simulink model "spot410"  (R2024b)
settings: Solver=ode4  StartTime=0.0  StopTime=tsim  FixedStep=baseRate  RelTol=1e-6  AbsTol=1e-6
values from neighbouring files (symbols this model uses):
  baseRate = paramEst(phase,coord).k2    [SpotEstimator.m]
undefined symbols (not defined in the file or in its folder): a1, a2, a3, b0, b1, b2, b3, dataRate, DiscIntNeverNeededParam, drop_states_ARM, drop_states_BLACK, drop_states_BLUE, drop_states_RED, F_black_X_nominal, F_black_Y_nominal, F_blue_X_nominal, F_blue_Y_nominal, F_red_X_nominal, F_red_Y_nominal, F_thrusters_BLACK, F_thrusters_BLUE, F_thrusters_RED, Gamma1_el, Gamma1_sh, Gamma1_wr, Gamma2_el, Gamma2_sh, Gamma2_wr, Gamma3_el, Gamma3_sh, Gamma3_wr, Gamma4_el, Gamma4_sh, Gamma4_wr, Gamma5_el, Gamma5_sh, Gamma5_wr, Gamma6_el, Gamma6_sh, Gamma6_wr, home_states_BLACK, home_states_BLUE, home_states_RED, IBLACK, IBLUE, IDIST, IEE, init_states_BLACK, init_states_BLUE, init_states_RED, IPROX, IRED, K_BLACK, K_BLUE, K_RED, Kd_elarm, Kd_sharm, Kd_tb, Kd_tblue, Kd_tr ... (+49)
libraries: simulink x30, nvidiaSharedBlocks x19, MainLibrary x5, dspinverses x3, nvidiaIMUSensorslib x1
(part 7 of 7)

== matlab function spot410/Simulate Plant Dynamics/RED and ARM Dynamics/RED + ARM/Inertia Function 1 ==
  data: mRED parameter; IRED parameter; Phi parameter; b0 parameter; a1 parameter; b1 parameter; a2 parameter; b2 parameter; a3 parameter; b3 parameter; mPROX parameter; mDIST parameter; mEE parameter; IPROX parameter; IDIST parameter; InertiaS output; x input; IEE parameter
function InertiaS = InertiaFunc3LINK(mRED, IRED, Phi, b0, a1, b1, a2, b2, a3, b3, mPROX, mDIST, mEE, IPROX, IDIST, x, IEE)

    q0 = x(3);
    q1 = x(4);
    q2 = x(5);
    q3 = x(6);
    
    t2 = a1+b1;
    t3 = a1.*mPROX;
    t4 = mDIST.*t2;
    t5 = mEE.*t2;
    t6 = q0+q1;
    t7 = cos(t6);
    t8 = t3+t4+t5;
    t9 = a2.*mDIST;
    t10 = a2+b2;
    t11 = mEE.*t10;
    t12 = q0+q1+q2;
    t13 = cos(t12);
    t14 = t9+t11;
    t15 = q0+q1+q2+q3;
    t16 = cos(t15);
    t17 = mRED+mPROX+mDIST+mEE;
    t18 = b0.*mPROX;
    t19 = b0.*mDIST;
    t20 = b0.*mEE;
    t21 = t18+t19+t20;
    t22 = (pi/2-Phi)+q0;
    t23 = sin(t6);
    t24 = sin(t12);
    t25 = sin(t15);
    t26 = a2.*mEE;
    t27 = b2.*mEE;
    t28 = t9+t26+t27;
    t29 = sin(t22);
    t86 = t7.*t8;
    t87 = t13.*t14;
    t88 = a3.*mEE.*t16;
    t30 = -t86-t87-t88-t21.*t29;
    t31 = cos(t22);
    t32 = t21.*t31;
    t89 = t8.*t23;
    t90 = t14.*t24;
    t91 = a3.*mEE.*t25;
    t33 = t32-t89-t90-t91;
    t34 = a1.^2;
    t35 = a2.^2;
    t36 = b0.^2;
    t37 = b1.^2;
    t38 = a1.*a2.*mDIST.*2.0;
    t39 = a1.*a2.*mEE.*2.0;
    t40 = a2.*b1.*mDIST.*2.0;
    t41 = a1.*b2.*mEE.*2.0;
    t42 = a2.*b1.*mEE.*2.0;
    t43 = b1.*b2.*mEE.*2.0;
    t44 = t38+t39+t40+t41+t42+t43;
    t45 = cos(q2);
    t46 = t44.*t45;
    t47 = a2.*a3.*mEE.*2.0;
    t48 = a3.*b2.*mEE.*2.0;
    t49 = t47+t48;
    t50 = cos(q3);
    t51 = t49.*t50;
    t52 = a1.*a3.*mEE.*2.0;
    t53 = a3.*b1.*mEE.*2.0;
    t54 = t52+t53;
    t55 = q2+q3;
    t56 = cos(t55);
    t57 = t54.*t56;
    t58 = (pi/2-Phi)-q1;
    t59 = sin(t58);
    t60 = -(pi/2-Phi)+q1+q2;
    t61 = sin(t60);
    t62 = -(pi/2-Phi)+q1+q2+q3;
    t63 = sin(t62);
    t64 = mPROX.*t34;
    t65 = mDIST.*t34;
    t66 = mEE.*t34;
    t67 = mDIST.*t35;
    t68 = mEE.*t35;
    t69 = a3.^2;
    t70 = mEE.*t69;
    t71 = mDIST.*t37;
    t72 = mEE.*t37;
    t73 = b2.^2;
    t74 = mEE.*t73;
    t75 = a1.*b1.*mDIST.*2.0;
    t76 = a1.*b1.*mEE.*2.0;
    t77 = a2.*b2.*mEE.*2.0;
    t78 = a2.*b0.*mDIST;
    t79 = a2.*b0.*mEE;
    t80 = b0.*b2.*mEE;
    t81 = t78+t79+t80;
    t82 = a1.*a3.*mEE;
    t83 = a3.*b1.*mEE;
    t84 = t82+t83;
    t85 = t56.*t84;
    t92 = a1.*b0.*mPROX;
    t93 = a1.*b0.*mDIST;
    t94 = a1.*b0.*mEE;
    t95 = b0.*b1.*mDIST;
    t96 = b0.*b1.*mEE;
    t97 = t92+t93+t94+t95+t96;
    t98 = t59.*t97;
    t112 = t61.*t81;
    t113 = a3.*b0.*mEE.*t63;
    t99 = IPROX+IDIST+IEE+t46+t51+t57+t64+t65+t66+t67+t68+t70+t71+t72+t74+t75+t76+t77+t98-t112-t113;
    t100 = a1.*a2.*mDIST;
    t101 = a1.*a2.*mEE;
    t102 = a2.*b1.*mDIST;
    t103 = a1.*b2.*mEE;
    t104 = a2.*b1.*mEE;
    t105 = b1.*b2.*mEE;
    t106 = t100+t101+t102+t103+t104+t105;
    t107 = t45.*t106;
    t108 = a2.*a3.*mEE;
    t109 = a3.*b2.*mEE;
    t110 = t108+t109;
    t111 = t50.*t110;
    t114 = IDIST+IEE+t51+t67+t68+t70+t74+t77+t85+t107;
    t115 = IEE+t70+t85+t111;
    t116 = IEE+t70+t111;
    InertiaS = reshape([t17,0.0,t30,-t86-t87-t88,-t88-t13.*t28,-t88,0.0,t17,t33,-t89-t90-t91,-t91-t24.*t28,-t91,t30,t33,IRED+IPROX+IDIST+IEE+t46+t51+t57+t64+t65+t66+t67+t68+t70+t71+t72+t74+t75+t76+t77+t59.*(a1.*b0.*mPROX.*2.0+a1.*b0.*mDIST.*2.0+a1.*b0.*mEE.*2.0+b0.*b1.*mDIST.*2.0+b0.*b1.*mEE.*2.0)+mPROX.*t36+mDIST.*t36+mEE.*t36-t61.*(a2.*b0.*mDIST.*2.0+a2.*b0.*mEE.*2.0+b0.*b2.*mEE.*2.0)-a3.*b0.*mEE.*t63.*2.0,t99,IDIST+IEE+t51+t67+t68+t70+t74+t77+t85+t107-t112-t113,IEE+t70+t85+t111-t113,-t7.*t8-t13.*t14-a3.*mEE.*t16,-t8.*t23-t14.*t24-a3.*mEE.*t25,t99,IPROX+IDIST+IEE+t46+t51+t57+t64+t65+t66+t67+t68+t70+t71+t72+t74+t75+t76+t77,t114,t115,-t13.*t28-a3.*mEE.*t16,-t24.*t28-a3.*mEE.*t25,IDIST+IEE+t51+t67+t68+t70+t74+t77+t85+t107-t61.*t81-a3.*b0.*mEE.*t63,t114,IDIST+IEE+t51+t67+t68+t70+t74+t77,t116,-a3.*mEE.*t16,-a3.*mEE.*t25,IEE+t70+t85+t111-a3.*b0.*mEE.*t63,t115,t116,IEE+t70],[6,6]);
end

== matlab function spot410/Simulate Plant Dynamics/BLUE Dynamics/Calculated & Store Measured States/Subsystem1/Enabled Subsystem/MATLAB Function ==
  data: y input; dy output; dt input; tau input; dy_prev input; ema_prev input; ema output
function [dy, ema] = realtime_derivative_ema(y, dt, tau, dy_prev, ema_prev)
    % Inputs:
    % y: Current measurement
    % dt: Time step
    % alpha: Smoothing factor (e.g., 0.1)

    alpha = 1 - exp(-dt / tau);
        
    % Update EMA
    ema = alpha.*y + (1 - alpha).*ema_prev;
    
    % Compute derivative
    dy = (ema - ema_prev)./dt;
    
end

== matlab function spot410/Simulate Plant Dynamics/BLACK Dynamics/Dynamics Model for BLACK/MATLAB Function ==
  data: control_inputs input; x_ddot output; mBLACK parameter; IBLACK parameter
function x_ddot = BLACK_dynamics(control_inputs, mBLACK, IBLACK)

%#codegen
% Fully define the size of x_ddot() for code generation:
x_ddot     = zeros(3,1);

% Extract the control inputs from the control_input vector:
Fx        = control_inputs(1);              % [N]
Fy        = control_inputs(2);              % [N]
Tz        = control_inputs(3);              % [N.m]

% Calculate the state acceleration vector:
x_ddot(1) = Fx/mBLACK;                      % [m/s^2]
x_ddot(2) = Fy/mBLACK;                      % [m/s^2]
x_ddot(3) = Tz/IBLACK;                      % [rad/s^2]

end

== matlab function spot410/Simulate Plant Dynamics/BLUE Dynamics/BLUE  Dynamics Model/MATLAB Function ==
  data: control_inputs input; x_ddot output; mBLUE parameter; IBLUE parameter
function x_ddot = BLUE_dynamics(control_inputs, mBLUE, IBLUE)%#codegen
% Fully define the size of x_ddot() for code generation:
x_ddot     = zeros(3,1);

% Extract the control inputs from the control_input vector:
Fx        = control_inputs(1);              % [N]
Fy        = control_inputs(2);              % [N]
Tz        = control_inputs(3);              % [N.m]

% Calculate the state acceleration vector:
x_ddot(1) = Fx/mBLUE;                      % [m/s^2]
x_ddot(2) = Fy/mBLUE;                      % [m/s^2]
x_ddot(3) = Tz/IBLUE;                      % [rad/s^2]

end

== matlab function spot410/Gyro.//Accel. Code/Log Gyro//Accel/Parse IMU Data ==
  data: WhoAmI input; RED_IMU_Ax output; IMU_Ax input; IMU_Ay input; IMU_Gz input; RED_IMU_Ay output; RED_IMU_Gz output; BLACK_IMU_Ax output; BLACK_IMU_Ay output; BLACK_IMU_Gz output; BLUE_IMU_Ax output; BLUE_IMU_Ay output; BLUE_IMU_Gz output
function [RED_IMU_Ax, RED_IMU_Ay, RED_IMU_Gz, BLACK_IMU_Ax, BLACK_IMU_Ay, BLACK_IMU_Gz, BLUE_IMU_Ax, BLUE_IMU_Ay, BLUE_IMU_Gz] = ParseIMUData(WhoAmI, IMU_Ax, IMU_Ay, IMU_Gz)

    if WhoAmI == 1 % This is RED

        RED_IMU_Ax = IMU_Ax;
        RED_IMU_Ay = IMU_Ay;
        RED_IMU_Gz = IMU_Gz;
        BLACK_IMU_Ax = 0;
        BLACK_IMU_Ay = 0;
        BLACK_IMU_Gz = 0;
        BLUE_IMU_Ax = 0;
        BLUE_IMU_Ay = 0;
        BLUE_IMU_Gz = 0;

    elseif WhoAmI == 2 % This is BLACK

        RED_IMU_Ax = 0;
        RED_IMU_Ay = 0;
        RED_IMU_Gz = 0;
        BLACK_IMU_Ax = IMU_Ax;
        BLACK_IMU_Ay = IMU_Ay;
        BLACK_IMU_Gz = IMU_Gz;
        BLUE_IMU_Ax = 0;
        BLUE_IMU_Ay = 0;
        BLUE_IMU_Gz = 0;

    elseif WhoAmI == 3 % This is BLUE

        RED_IMU_Ax = 0;
        RED_IMU_Ay = 0;
        RED_IMU_Gz = 0;
        BLACK_IMU_Ax = 0;
        BLACK_IMU_Ay = 0;
        BLACK_IMU_Gz = 0;
        BLUE_IMU_Ax = IMU_Ax;
        BLUE_IMU_Ay = IMU_Ay;
        BLUE_IMU_Gz = IMU_Gz;

    else 

        RED_IMU_Ax = 0;
        RED_IMU_Ay = 0;
        RED_IMU_Gz = 0;
        BLACK_IMU_Ax = 0;
        BLACK_IMU_Ay = 0;
        BLACK_IMU_Gz = 0;
        BLUE_IMU_Ax = 0;
        BLUE_IMU_Ay = 0;
        BLUE_IMU_Gz = 0;       

    end

end

== matlab function spot410/Simulate Plant Dynamics/BLUE Dynamics/Calculated & Store Measured States/Subsystem2/Enabled Subsystem/MATLAB Function ==
  data: y input; dy output; dt input; tau input; dy_prev input; ema_prev input; ema output
function [dy, ema] = realtime_derivative_ema(y, dt, tau, dy_prev, ema_prev)
    % Inputs:
    % y: Current measurement
    % dt: Time step
    % alpha: Smoothing factor (e.g., 0.1)

    alpha = 1 - exp(-dt / tau);
        
    % Update EMA
    ema = alpha.*y + (1 - alpha).*ema_prev;
    
    % Compute derivative
    dy = (ema - ema_prev)./dt;
    
end

== matlab function spot410/Simulate Plant Dynamics/BLUE Dynamics/Data @ Measurement Rate/Calculate True Time Step/MATLAB Function ==
  data: dt input; dt_out output; dataRate input
function dt_out = CheckforInvalidTime(dt, dataRate)

    if dt <= 0

        dt_out = dataRate;

    else

        dt_out = dt;

    end


end

== matlab function spot410/SpotGnc/SpotCtrlErr ==
  data: phase input; ref input; ref_vel input; est input; est_vel input; err output; paramCtrlErr parameter; err_vel output
function [err,err_vel] = SpotCtrlErr(phase, ref, ref_vel, est, est_vel, paramCtrlErr)

    [err,err_vel] = SpotCtrlErr(phase, ref, ref_vel, est, est_vel, paramCtrlErr);

end

== matlab function spot410/PhaseSpace Camera Code/Use Hardware to Obtain States/Store RED Data/Subsystem2/Enabled Subsystem/MATLAB Function ==
  data: y input; dy output; dt input; tau input; dy_prev input; ema_prev input; ema output
function [dy, ema] = realtime_derivative_ema(y, dt, tau, dy_prev, ema_prev)
    % Inputs:
    % y: Current measurement
    % dt: Time step
    % alpha: Smoothing factor (e.g., 0.1)

    alpha = 1 - exp(-dt / tau);
        
    % Update EMA
    ema = alpha.*y + (1 - alpha).*ema_prev;
    
    % Compute derivative
    dy = (ema - ema_prev)./dt;
    
end

== matlab function spot410/PhaseSpace Camera Code/Use Hardware to Obtain States/Store BLACK Data/Calculate True Time Step/MATLAB Function ==
  data: dt input; dt_out output; dataRate input
function dt_out = CheckforInvalidTime(dt, dataRate)

    if dt <= 0

        dt_out = dataRate;

    else

        dt_out = dt;

    end


end

== matlab function spot410/PhaseSpace Camera Code/Use Hardware to Obtain States/Store RED Data/Calculate True Time Step/MATLAB Function ==
  data: dt input; dt_out output; dataRate input
function dt_out = CheckforInvalidTime(dt, dataRate)

    if dt <= 0

        dt_out = dataRate;

    else

        dt_out = dt;

    end


end

== matlab function spot410/PhaseSpace Camera Code/Use Hardware to Obtain States/Store BLACK Data/Subsystem1/Enabled Subsystem/MATLAB Function ==
  data: y input; dy output; dt input; tau input; dy_prev input; ema_prev input; ema output
function [dy, ema] = realtime_derivative_ema(y, dt, tau, dy_prev, ema_prev)
    % Inputs:
    % y: Current measurement
    % dt: Time step
    % alpha: Smoothing factor (e.g., 0.1)

    alpha = 1 - exp(-dt / tau);
        
    % Update EMA
    ema = alpha.*y + (1 - alpha).*ema_prev;
    
    % Compute derivative
    dy = (ema - ema_prev)./dt;
    
end

== matlab function spot410/PhaseSpace Camera Code/Use Hardware to Obtain States/Store BLACK Data/Subsystem2/Enabled Subsystem/MATLAB Function ==
  data: y input; dy output; dt input; tau input; dy_prev input; ema_prev input; ema output
function [dy, ema] = realtime_derivative_ema(y, dt, tau, dy_prev, ema_prev)
    % Inputs:
    % y: Current measurement
    % dt: Time step
    % alpha: Smoothing factor (e.g., 0.1)

    alpha = 1 - exp(-dt / tau);
        
    % Update EMA
    ema = alpha.*y + (1 - alpha).*ema_prev;
    
    % Compute derivative
    dy = (ema - ema_prev)./dt;
    
end

== matlab function spot410/PhaseSpace Camera Code/Use Hardware to Obtain States/Store BLUE Data/Calculate True Time Step/MATLAB Function ==
  data: dt input; dt_out output; dataRate input
function dt_out = CheckforInvalidTime(dt, dataRate)

    if dt <= 0

        dt_out = dataRate;

    else

        dt_out = dt;

    end


end

== matlab function spot410/PhaseSpace Camera Code/Use Hardware to Obtain States/Store BLUE Data/Subsystem1/Enabled Subsystem/MATLAB Function ==
  data: y input; dy output; dt input; tau input; dy_prev input; ema_prev input; ema output
function [dy, ema] = realtime_derivative_ema(y, dt, tau, dy_prev, ema_prev)
    % Inputs:
    % y: Current measurement
    % dt: Time step
    % alpha: Smoothing factor (e.g., 0.1)

    alpha = 1 - exp(-dt / tau);
        
    % Update EMA
    ema = alpha.*y + (1 - alpha).*ema_prev;
    
    % Compute derivative
    dy = (ema - ema_prev)./dt;
    
end

== matlab function spot410/PhaseSpace Camera Code/Use Hardware to Obtain States/Store BLUE Data/Subsystem2/Enabled Subsystem/MATLAB Function ==
  data: y input; dy output; dt input; tau input; dy_prev input; ema_prev input; ema output
function [dy, ema] = realtime_derivative_ema(y, dt, tau, dy_prev, ema_prev)
    % Inputs:
    % y: Current measurement
    % dt: Time step
    % alpha: Smoothing factor (e.g., 0.1)

    alpha = 1 - exp(-dt / tau);
        
    % Update EMA
    ema = alpha.*y + (1 - alpha).*ema_prev;
    
    % Compute derivative
    dy = (ema - ema_prev)./dt;
    
end

== matlab function spot410/Simulate Plant Dynamics/RED and ARM Dynamics/RED Only/Dynamics Model for RED/MATLAB Function ==
  data: control_inputs input; x_ddot output; mRED parameter; IRED parameter

    function x_ddot = RED_dynamics(control_inputs, mRED, IRED)

        %#codegen
        % Fully define the size of x_ddot() for code generation:
        x_ddot     = zeros(3,1);

        % Extract the servicer model parameters from the model_param vector defined
        % in initialize.m:

        % Extract the control inputs from the control_input vector:
        Fx        = control_inputs(1);              % [N]
        Fy        = control_inputs(2);              % [N]
        Tz        = control_inputs(3);              % [N.m]

        % Calculate the state acceleration vector:
        x_ddot(1) = Fx/mRED;                      % [m/s^2]
        x_ddot(2) = Fy/mRED;                      % [m/s^2]
        x_ddot(3) = Tz/IRED;                      % [rad/s^2]

    end

== matlab function spot410/SpotGnc/SpotMeasProc ==
  data: phase input; meas input; proc output; paramMeasProc parameter
function proc  = SpotMeasProc(phase, meas, paramMeasProc)

    [proc] = SpotMeasProc(phase, meas, paramMeasProc);

end

== matlab function spot410/Simulate Plant Dynamics/RED and ARM Dynamics/RED + ARM/Data @ Measurement Rate/Calculate True Time Step/MATLAB Function ==
  data: dt input; dt_out output; dataRate input
function dt_out = CheckforInvalidTime(dt, dataRate)

    if dt <= 0

        dt_out = dataRate;

    else

        dt_out = dt;

    end


end

== matlab function spot410/Simulate Plant Dynamics/RED and ARM Dynamics/RED + ARM/Calculated & Store Measured States/Subsystem3/Enabled Subsystem/MATLAB Function ==
  data: y input; dy output; dt input; tau input; dy_prev input; ema_prev input; ema output
function [dy, ema] = realtime_derivative_ema(y, dt, tau, dy_prev, ema_prev)
    % Inputs:
    % y: Current measurement
    % dt: Time step
    % alpha: Smoothing factor (e.g., 0.1)

    alpha = 1 - exp(-dt / tau);
        
    % Update EMA
    ema = alpha.*y + (1 - alpha).*ema_prev;
    
    % Compute derivative
    dy = (ema - ema_prev)./dt;
    
end

== matlab function spot410/Simulate Plant Dynamics/RED and ARM Dynamics/RED + ARM/Calculated & Store Measured States/Subsystem4/Enabled Subsystem/MATLAB Function ==
  data: y input; dy output; dt input; tau input; dy_prev input; ema_prev input; ema output
function [dy, ema] = realtime_derivative_ema(y, dt, tau, dy_prev, ema_prev)
    % Inputs:
    % y: Current measurement
    % dt: Time step
    % alpha: Smoothing factor (e.g., 0.1)

    alpha = 1 - exp(-dt / tau);
        
    % Update EMA
    ema = alpha.*y + (1 - alpha).*ema_prev;
    
    % Compute derivative
    dy = (ema - ema_prev)./dt;
    
end

== matlab function spot410/Simulate Plant Dynamics/RED and ARM Dynamics/RED + ARM/Calculated & Store Measured States/Subsystem5/Enabled Subsystem/MATLAB Function ==
  data: y input; dy output; dt input; tau input; dy_prev input; ema_prev input; ema output
function [dy, ema] = realtime_derivative_ema(y, dt, tau, dy_prev, ema_prev)
    % Inputs:
    % y: Current measurement
    % dt: Time step
    % alpha: Smoothing factor (e.g., 0.1)

    alpha = 1 - exp(-dt / tau);
        
    % Update EMA
    ema = alpha.*y + (1 - alpha).*ema_prev;
    
    % Compute derivative
    dy = (ema - ema_prev)./dt;
    
end

== matlab function spot410/Thruster Control Code/Change BLACK Behavior/Calculate Duty Cycle/Generate Initial Guess/MATLAB Function ==
  data: H output; thruster_dist2CG_BLACK parameter; F_thrusters_BLACK parameter
function H = MakeH(thruster_dist2CG_BLACK,F_thrusters_BLACK)

    Vec1 = [ -1
             -1
              0 
              0
              1
              1
              0
              0 ];
          
    Vec2 = [  0
              0
              1
              1
              0
              0
             -1
             -1 ];
         
    Vec3 = thruster_dist2CG_BLACK./1000;
    
    Mat1 = [Vec1, Vec2, Vec3]';
    
    Mat2 = diag((F_thrusters_BLACK./2));
    
    H    = Mat1*Mat2;

end

== matlab function spot410/Thruster Control Code/Change BLACK Behavior/Calculate Duty Cycle/MATLAB Function5 ==
  data: H_final output; u_desired input; duty_cycles output; x0 input; thruster_dist2CG_BLACK parameter; F_black_X_nominal parameter; F_black_Y_nominal parameter; max_iters parameter; tol parameter
function [H_final,duty_cycles] = optimize_duty_cycle_with_decay(u_desired, x0, thruster_dist2CG_BLACK, F_black_X_nominal, F_black_Y_nominal, max_iters, tol)
    % Optimizes thruster duty cycles with decay factor updates
    %
    % Inputs:
    %   u_desired - Desired force and torque vector [Fx; Fy; M] (3x1)
    %   x0 - Initial guess for duty cycles (vector, 8x1)
    %   max_iters - Maximum number of iterations for convergence
    %   tol - Convergence tolerance for duty cycles
    %   thruster_dist2CG_BLACK - Distances of thrusters from CG (vector, mm)
    %   F_red_X_nominal - Nominal X thruster force (scalar, N)
    %   F_red_Y_nominal - Nominal Y thruster force (scalar, N)
    %
    % Outputs:
    %   duty_cycles - Optimal duty cycles for each thruster (vector, 8x1)

    % Initialization
    num_thrusters = length(x0);
    duty_cycles = x0; % Start with the initial guess
    thrust_decay_factor = 1; % Initial decay factor
    prev_duty_cycles = duty_cycles + 2 * tol; % Ensure loop starts

    % Iterative optimization process
    for iter = 1:max_iters
        % Update H matrix based on the current decay factor
        H = MakeHWithDecay(thruster_dist2CG_BLACK, F_black_X_nominal, thrust_decay_factor, F_black_Y_nominal);
        
        % Define quadratic programming problem
        Q = 2 * (H' * H); % Quadratic term
        c = -2 * (H' * u_desired); % Linear term
        lb = zeros(num_thrusters, 1); % Lower bounds
        ub = ones(num_thrusters, 1); % Upper bounds
        options = optimoptions('quadprog', 'Display', 'off', 'Algorithm', 'active-set', 'MaxIterations', 5);
        
        % Solve for optimal duty cycles
        [duty_cycles, ~, ~] = quadprog(Q, c, [], [], [], [], lb, ub, duty_cycles, options);
        
        % Update decay factor based on the current duty cycles
        [thrust_decay_factor, ~] = check_thrust_decay(duty_cycles);
                
        % Check convergence criteria
        if norm(duty_cycles - prev_duty_cycles, Inf) < tol
            H_final = MakeHWithDecayRecalculateForce(thruster_dist2CG_BLACK, F_black_X_nominal, thrust_decay_factor, F_black_Y_nominal);
            return;
        end
            
        
        % Update for next iteration
        prev_duty_cycles = duty_cycles;
    end
    
    H_final = MakeHWithDecayRecalculateForce(thruster_dist2CG_BLACK, F_black_X_nominal, thrust_decay_factor, F_black_Y_nominal);
   

end

function H = MakeHWithDecay(thruster_dist2CG, F_X_nominal, thrust_decay_factor, F_Y_nominal)
    % Constructs the H matrix with thrust decay adjustments
    %
    % Inputs:
    %   thruster_dist2CG - Distances of thrusters from CG (vector, mm)
    %   F_X_nominal - Nominal X thruster force (scalar, N)
    %   thrust_decay_factor - Decay factor for thrust (scalar)
    %   F_Y_nominal - Nominal Y thruster force (scalar, N)
    %
    % Output:
    %   H - H matrix for optimization (3x8)

    % Adjust thruster distances (convert to meters)
    adjusted_thruster_dist2CG = thruster_dist2CG / 1000;

    % Define thruster contribution vectors
    Vec1 = [-1; -1;  0;  0;  1;  1;  0;  0]; % X-component
    Vec2 = [ 0;  0;  1;  1;  0;  0; -1; -1]; % Y-component
    Vec3 = adjusted_thruster_dist2CG;        % Moment arm (Z)

    % Combine vectors into the H matrix structure
    Mat1 = [Vec1, Vec2, Vec3]';
    
    % Adjust thruster forces with decay factor
    F_thrusters = [F_X_nominal; F_X_nominal; F_Y_nominal; F_Y_nominal; 
                   F_X_nominal; F_X_nominal; F_Y_nominal; F_Y_nominal] * thrust_decay_factor;

    % Scale forces for H matrix
    Mat2 = diag(F_thrusters / 2);

    % Compute final H matrix
    H = Mat1 * Mat2;
end

function H = MakeHWithDecayRecalculateForce(thruster_dist2CG, F_X_nominal, thrust_decay_factor, F_Y_nominal)
    % Constructs the H matrix with thrust decay adjustments
    %
    % Inputs:
    %   thruster_dist2CG - Distances of thrusters from CG (vector, mm)
    %   F_X_nominal - Nominal X thruster force (scalar, N)
    %   thrust_decay_factor - Decay factor for thrust (scalar)
    %   F_Y_nominal - Nominal Y thruster force (scalar, N)
    %
    % Output:
    %   H - H matrix for optimization (3x8)

    % Adjust thruster distances (convert to meters)
    adjusted_thruster_dist2CG = thruster_dist2CG / 1000;

    % Define thruster contribution vectors
    Vec1 = [-1; -1;  0;  0;  1;  1;  0;  0]; % X-component
    Vec2 = [ 0;  0;  1;  1;  0;  0; -1; -1]; % Y-component
    Vec3 = adjusted_thruster_dist2CG;        % Moment arm (Z)

    % Combine vectors into the H matrix structure
    Mat1 = [Vec1, Vec2, Vec3]';
    
    % Adjust thruster forces with decay factor
    F_thrusters = [F_X_nominal; F_X_nominal; F_Y_nominal; F_Y_nominal; 
                   F_X_nominal; F_X_nominal; F_Y_nominal; F_Y_nominal] * thrust_decay_factor;

    % Scale forces for H matrix
    Mat2 = diag(F_thrusters);

    % Compute final H matrix
    H = Mat1 * Mat2;
end

function [thrust_decay_factor, count] = check_thrust_decay(PWMs)
    % Updates the thrust decay factor based on current duty cycles
    %
    % Inputs:
    %   PWMs - Current duty cycle values (vector)
    %
    % Outputs:
    %   thrust_decay_factor - Updated decay factor (scalar)
    %   count - Number of active thrusters (scalar)

    % Normalize PWMs if necessary
    if max(PWMs) > 1
        PWMs = PWMs / max(PWMs);
    end

    % Count active thrusters
    count = sum(PWMs > 0);
    
    % Compute average duty cycle for active thrusters
    average_duty_cycle_per_thruster = sum(max(PWMs, 0)) / max(count, 1);

    % Update thrust decay factor based on average duty cycle
    if average_duty_cycle_per_thruster < 0.3 || count == 0
        thrust_decay_factor = 1;
    else
        thrust_decay_factor = max(0.6 - 2 * average_duty_cycle_per_thruster + 1, 0.5);
    end
end

== matlab function spot410/Thruster Control Code/Change BLACK Behavior/Calculate Duty Cycle/Rotate Forces to Inertial/Create Rotation Matrix ==
  data: Rz input; C_Ib output
function C_Ib = RotateFrame(Rz)

C_bI = [  cos(Rz) sin(Rz)
         -sin(Rz) cos(Rz) ];

C_Ib = inv(C_bI);

end

== matlab function spot410/Thruster Control Code/Change BLACK Behavior/Rotate Forces to Body/Create Rotation Matrix ==
  data: Rz input; C_bI output
function C_bI = RotateFrame(Rz)

C_bI = [  cos(Rz) sin(Rz)
         -sin(Rz) cos(Rz) ];

end

== matlab function spot410/Thruster Control Code/Change BLUE Behavior/Calculate Duty Cycle/Generate Initial Guess/MATLAB Function ==
  data: H output; thruster_dist2CG_BLUE parameter; F_thrusters_BLUE parameter
function H = MakeH(thruster_dist2CG_BLUE,F_thrusters_BLUE)

    Vec1 = [ -1
             -1
              0 
              0
              1
              1
              0
              0 ];
          
    Vec2 = [  0
              0
              1
              1
              0
              0
             -1
             -1 ];
         
    Vec3 = thruster_dist2CG_BLUE./1000;
    
    Mat1 = [Vec1, Vec2, Vec3]';
    
    Mat2 = diag((F_thrusters_BLUE./2));
    
    H    = Mat1*Mat2;

end

== matlab function spot410/Thruster Control Code/Change BLUE Behavior/Calculate Duty Cycle/MATLAB Function5 ==
  data: H_final output; u_desired input; duty_cycles output; x0 input; thruster_dist2CG_BLUE parameter; F_blue_X_nominal parameter; F_blue_Y_nominal parameter; max_iters parameter; tol parameter
function [H_final,duty_cycles] = optimize_duty_cycle_with_decay(u_desired, x0, thruster_dist2CG_BLUE, F_blue_X_nominal, F_blue_Y_nominal, max_iters, tol)
    % Optimizes thruster duty cycles with decay factor updates
    %
    % Inputs:
    %   u_desired - Desired force and torque vector [Fx; Fy; M] (3x1)
    %   x0 - Initial guess for duty cycles (vector, 8x1)
    %   max_iters - Maximum number of iterations for convergence
    %   tol - Convergence tolerance for duty cycles
    %   thruster_dist2CG_BLUE - Distances of thrusters from CG (vector, mm)
    %   F_red_X_nominal - Nominal X thruster force (scalar, N)
    %   F_red_Y_nominal - Nominal Y thruster force (scalar, N)
    %
    % Outputs:
    %   duty_cycles - Optimal duty cycles for each thruster (vector, 8x1)

    % Initialization
    num_thrusters = length(x0);
    duty_cycles = x0; % Start with the initial guess
    thrust_decay_factor = 1; % Initial decay factor
    prev_duty_cycles = duty_cycles + 2 * tol; % Ensure loop starts

    % Iterative optimization process
    for iter = 1:max_iters
        % Update H matrix based on the current decay factor
        H = MakeHWithDecay(thruster_dist2CG_BLUE, F_blue_X_nominal, thrust_decay_factor, F_blue_Y_nominal);
        
        % Define quadratic programming problem
        Q = 2 * (H' * H); % Quadratic term
        c = -2 * (H' * u_desired); % Linear term
        lb = zeros(num_thrusters, 1); % Lower bounds
        ub = ones(num_thrusters, 1); % Upper bounds
        options = optimoptions('quadprog', 'Display', 'off', 'Algorithm', 'active-set', 'MaxIterations', 5);
        
        % Solve for optimal duty cycles
        [duty_cycles, ~, ~] = quadprog(Q, c, [], [], [], [], lb, ub, duty_cycles, options);
        
        % Update decay factor based on the current duty cycles
        [thrust_decay_factor, ~] = check_thrust_decay(duty_cycles);
                
        % Check convergence criteria
        if norm(duty_cycles - prev_duty_cycles, Inf) < tol
            H_final = MakeHWithDecayRecalculateForce(thruster_dist2CG_BLUE, F_blue_X_nominal, thrust_decay_factor, F_blue_Y_nominal);
            return;
        end
            
        
        % Update for next iteration
        prev_duty_cycles = duty_cycles;
    end
    
    H_final = MakeHWithDecayRecalculateForce(thruster_dist2CG_BLUE, F_blue_X_nominal, thrust_decay_factor, F_blue_Y_nominal);
   

end

function H = MakeHWithDecay(thruster_dist2CG, F_X_nominal, thrust_decay_factor, F_Y_nominal)
    % Constructs the H matrix with thrust decay adjustments
    %
    % Inputs:
    %   thruster_dist2CG - Distances of thrusters from CG (vector, mm)
    %   F_X_nominal - Nominal X thruster force (scalar, N)
    %   thrust_decay_factor - Decay factor for thrust (scalar)
    %   F_Y_nominal - Nominal Y thruster force (scalar, N)
    %
    % Output:
    %   H - H matrix for optimization (3x8)

    % Adjust thruster distances (convert to meters)
    adjusted_thruster_dist2CG = thruster_dist2CG / 1000;

    % Define thruster contribution vectors
    Vec1 = [-1; -1;  0;  0;  1;  1;  0;  0]; % X-component
    Vec2 = [ 0;  0;  1;  1;  0;  0; -1; -1]; % Y-component
    Vec3 = adjusted_thruster_dist2CG;        % Moment arm (Z)

    % Combine vectors into the H matrix structure
    Mat1 = [Vec1, Vec2, Vec3]';
    
    % Adjust thruster forces with decay factor
    F_thrusters = [F_X_nominal; F_X_nominal; F_Y_nominal; F_Y_nominal; 
                   F_X_nominal; F_X_nominal; F_Y_nominal; F_Y_nominal] * thrust_decay_factor;

    % Scale forces for H matrix
    Mat2 = diag(F_thrusters / 2);

    % Compute final H matrix
    H = Mat1 * Mat2;
end

function H = MakeHWithDecayRecalculateForce(thruster_dist2CG, F_X_nominal, thrust_decay_factor, F_Y_nominal)
    % Constructs the H matrix with thrust decay adjustments
    %
    % Inputs:
    %   thruster_dist2CG - Distances of thrusters from CG (vector, mm)
    %   F_X_nominal - Nominal X thruster force (scalar, N)
    %   thrust_decay_factor - Decay factor for thrust (scalar)
    %   F_Y_nominal - Nominal Y thruster force (scalar, N)
    %
    % Output:
    %   H - H matrix for optimization (3x8)

    % Adjust thruster distances (convert to meters)
    adjusted_thruster_dist2CG = thruster_dist2CG / 1000;

    % Define thruster contribution vectors
    Vec1 = [-1; -1;  0;  0;  1;  1;  0;  0]; % X-component
    Vec2 = [ 0;  0;  1;  1;  0;  0; -1; -1]; % Y-component
    Vec3 = adjusted_thruster_dist2CG;        % Moment arm (Z)

    % Combine vectors into the H matrix structure
    Mat1 = [Vec1, Vec2, Vec3]';
    
    % Adjust thruster forces with decay factor
    F_thrusters = [F_X_nominal; F_X_nominal; F_Y_nominal; F_Y_nominal; 
                   F_X_nominal; F_X_nominal; F_Y_nominal; F_Y_nominal] * thrust_decay_factor;

    % Scale forces for H matrix
    Mat2 = diag(F_thrusters);

    % Compute final H matrix
    H = Mat1 * Mat2;
end

function [thrust_decay_factor, count] = check_thrust_decay(PWMs)
    % Updates the thrust decay factor based on current duty cycles
    %
    % Inputs:
    %   PWMs - Current duty cycle values (vector)
    %
    % Outputs:
    %   thrust_decay_factor - Updated decay factor (scalar)
    %   count - Number of active thrusters (scalar)

    % Normalize PWMs if necessary
    if max(PWMs) > 1
        PWMs = PWMs / max(PWMs);
    end

    % Count active thrusters
    count = sum(PWMs > 0);
    
    % Compute average duty cycle for active thrusters
    average_duty_cycle_per_thruster = sum(max(PWMs, 0)) / max(count, 1);

    % Update thrust decay factor based on average duty cycle
    if average_duty_cycle_per_thruster < 0.3 || count == 0
        thrust_decay_factor = 1;
    else
        thrust_decay_factor = max(0.6 - 2 * average_duty_cycle_per_thruster + 1, 0.5);
    end
end

== matlab function spot410/Thruster Control Code/Change BLUE Behavior/Calculate Duty Cycle/Rotate Forces to Inertial/Create Rotation Matrix ==
  data: Rz input; C_Ib output
function C_Ib = RotateFrame(Rz)

C_bI = [  cos(Rz) sin(Rz)
         -sin(Rz) cos(Rz) ];

C_Ib = inv(C_bI);

end

== matlab function spot410/2 - Guidance/Default APF PPL (BLACK)/MATLAB Function ==
  data: desiredPosition input; currentPosition output; currentPosition input; obstacles input; attractiveGain input; repulsiveGain input; influenceRange input; angularGain input; baseRate parameter
function currentPosition = APFPathPlanner(desiredPosition, currentPosition, obstacles, attractiveGain, repulsiveGain, influenceRange, angularGain, baseRate)
    % APFPathPlanner for real-time path planning in Simulink
    % Controls X, Y, and Attitude (Theta)
    % currentPosition: [x, y, theta]
    % desiredPosition: [x, y, theta]
    % obstacles: Nx2 matrix of obstacle positions [x, y]
    % attractiveGain: Scalar for attractive force
    % repulsiveGain: Scalar for repulsive force
    % influenceRange: Scalar, range for obstacle influence
    % angularGain: Scalar for angular adjustment


    % Position control for X and Y
    attractiveForce = attractiveGain * (desiredPosition(1:2) - currentPosition(1:2));
    repulsiveForce = zeros(1, 2);

    % % Repulsive force from obstacles
    for i = 1:size(obstacles, 1)
        obstaclePos = obstacles(i, :);
        distanceToObstacle = norm(currentPosition(1:2) - obstaclePos);

        if distanceToObstacle < influenceRange
            directionFromObstacle = (currentPosition(1:2) - obstaclePos) / distanceToObstacle;
            magnitude = repulsiveGain * (1 / distanceToObstacle - 1 / influenceRange) * (1 / distanceToObstacle^2);
            repulsiveForce = repulsiveForce + magnitude * directionFromObstacle;
        end
    end

    % Combine attractive and repulsive forces
    totalForce = attractiveForce + repulsiveForce;

    % Update X and Y position
    deltaT = baseRate;
    newPosition = currentPosition(1:2) + deltaT * totalForce;

    % Attitude control for Theta
    angularDifference = atan2(sin(desiredPosition(3) - currentPosition(3)), cos(desiredPosition(3) - currentPosition(3)));
    newTheta = currentPosition(3) + angularGain * angularDifference * deltaT;

    % Normalize newTheta to be within -pi to pi
    newTheta = atan2(sin(newTheta), cos(newTheta));

    % Update currentPosition with new position and attitude
    currentPosition = [newPosition, newTheta];

end

== matlab function spot410/Thruster Control Code/Change BLUE Behavior/Rotate Forces to Body/Create Rotation Matrix ==
  data: Rz input; C_bI output
function C_bI = RotateFrame(Rz)

C_bI = [  cos(Rz) sin(Rz)
         -sin(Rz) cos(Rz) ];

end

== matlab function spot410/Thruster Control Code/Change RED Behavior/Calculate Duty Cycle/Generate Initial Guess/MATLAB Function ==
  data: H output; thruster_dist2CG_RED parameter; F_thrusters_RED parameter
function H = MakeH(thruster_dist2CG_RED,F_thrusters_RED)

    Vec1 = [ -1
             -1
              0 
              0
              1
              1
              0
              0 ];
          
    Vec2 = [  0
              0
              1
              1
              0
              0
             -1
             -1 ];
         
    Vec3 = thruster_dist2CG_RED./1000;
    
    Mat1 = [Vec1, Vec2, Vec3]';
    
    Mat2 = diag((F_thrusters_RED./2));
    
    H    = Mat1*Mat2;

end

== matlab function spot410/Thruster Control Code/Change RED Behavior/Calculate Duty Cycle/MATLAB Function5 ==
  data: H_final output; u_desired input; duty_cycles output; x0 input; thruster_dist2CG_RED parameter; F_red_X_nominal parameter; F_red_Y_nominal parameter; max_iters parameter; tol parameter
function [H_final,duty_cycles] = optimize_duty_cycle_with_decay(u_desired, x0, thruster_dist2CG_RED, F_red_X_nominal, F_red_Y_nominal, max_iters, tol)
    % Optimizes thruster duty cycles with decay factor updates
    %
    % Inputs:
    %   u_desired - Desired force and torque vector [Fx; Fy; M] (3x1)
    %   x0 - Initial guess for duty cycles (vector, 8x1)
    %   max_iters - Maximum number of iterations for convergence
    %   tol - Convergence tolerance for duty cycles
    %   thruster_dist2CG_RED - Distances of thrusters from CG (vector, mm)
    %   F_red_X_nominal - Nominal X thruster force (scalar, N)
    %   F_red_Y_nominal - Nominal Y thruster force (scalar, N)
    %
    % Outputs:
    %   duty_cycles - Optimal duty cycles for each thruster (vector, 8x1)

    % Initialization
    num_thrusters = length(x0);
    duty_cycles = x0; % Start with the initial guess
    thrust_decay_factor = 1; % Initial decay factor
    prev_duty_cycles = duty_cycles + 2 * tol; % Ensure loop starts

    % Iterative optimization process
    for iter = 1:max_iters
        % Update H matrix based on the current decay factor
        H = MakeHWithDecay(thruster_dist2CG_RED, F_red_X_nominal, thrust_decay_factor, F_red_Y_nominal);
        
        % Define quadratic programming problem
        Q = 2 * (H' * H); % Quadratic term
        c = -2 * (H' * u_desired); % Linear term
        lb = zeros(num_thrusters, 1); % Lower bounds
        ub = ones(num_thrusters, 1); % Upper bounds
        options = optimoptions('quadprog', 'Display', 'off', 'Algorithm', 'active-set', 'MaxIterations', 5);
        
        % Solve for optimal duty cycles
        [duty_cycles, ~, ~] = quadprog(Q, c, [], [], [], [], lb, ub, duty_cycles, options);
        
        % Update decay factor based on the current duty cycles
        [thrust_decay_factor, ~] = check_thrust_decay(duty_cycles);
                
        % Check convergence criteria
        if norm(duty_cycles - prev_duty_cycles, Inf) < tol
            H_final = MakeHWithDecayRecalculateForce(thruster_dist2CG_RED, F_red_X_nominal, thrust_decay_factor, F_red_Y_nominal);
            return;
        end
            
        
        % Update for next iteration
        prev_duty_cycles = duty_cycles;
    end
    
    H_final = MakeHWithDecayRecalculateForce(thruster_dist2CG_RED, F_red_X_nominal, thrust_decay_factor, F_red_Y_nominal);
   

end

function H = MakeHWithDecay(thruster_dist2CG, F_X_nominal, thrust_decay_factor, F_Y_nominal)
    % Constructs the H matrix with thrust decay adjustments
    %
    % Inputs:
    %   thruster_dist2CG - Distances of thrusters from CG (vector, mm)
    %   F_X_nominal - Nominal X thruster force (scalar, N)
    %   thrust_decay_factor - Decay factor for thrust (scalar)
    %   F_Y_nominal - Nominal Y thruster force (scalar, N)
    %
    % Output:
    %   H - H matrix for optimization (3x8)

    % Adjust thruster distances (convert to meters)
    adjusted_thruster_dist2CG = thruster_dist2CG / 1000;

    % Define thruster contribution vectors
    Vec1 = [-1; -1;  0;  0;  1;  1;  0;  0]; % X-component
    Vec2 = [ 0;  0;  1;  1;  0;  0; -1; -1]; % Y-component
    Vec3 = adjusted_thruster_dist2CG;        % Moment arm (Z)

    % Combine vectors into the H matrix structure
    Mat1 = [Vec1, Vec2, Vec3]';
    
    % Adjust thruster forces with decay factor
    F_thrusters = [F_X_nominal; F_X_nominal; F_Y_nominal; F_Y_nominal; 
                   F_X_nominal; F_X_nominal; F_Y_nominal; F_Y_nominal] * thrust_decay_factor;

    % Scale forces for H matrix
    Mat2 = diag(F_thrusters / 2);

    % Compute final H matrix
    H = Mat1 * Mat2;
end

function H = MakeHWithDecayRecalculateForce(thruster_dist2CG, F_X_nominal, thrust_decay_factor, F_Y_nominal)
    % Constructs the H matrix with thrust decay adjustments
    %
    % Inputs:
    %   thruster_dist2CG - Distances of thrusters from CG (vector, mm)
    %   F_X_nominal - Nominal X thruster force (scalar, N)
    %   thrust_decay_factor - Decay factor for thrust (scalar)
    %   F_Y_nominal - Nominal Y thruster force (scalar, N)
    %
    % Output:
    %   H - H matrix for optimization (3x8)

    % Adjust thruster distances (convert to meters)
    adjusted_thruster_dist2CG = thruster_dist2CG / 1000;

    % Define thruster contribution vectors
    Vec1 = [-1; -1;  0;  0;  1;  1;  0;  0]; % X-component
    Vec2 = [ 0;  0;  1;  1;  0;  0; -1; -1]; % Y-component
    Vec3 = adjusted_thruster_dist2CG;        % Moment arm (Z)

    % Combine vectors into the H matrix structure
    Mat1 = [Vec1, Vec2, Vec3]';
    
    % Adjust thruster forces with decay factor
    F_thrusters = [F_X_nominal; F_X_nominal; F_Y_nominal; F_Y_nominal; 
                   F_X_nominal; F_X_nominal; F_Y_nominal; F_Y_nominal] * thrust_decay_factor;

    % Scale forces for H matrix
    Mat2 = diag(F_thrusters);

    % Compute final H matrix
    H = Mat1 * Mat2;
end

function [thrust_decay_factor, count] = check_thrust_decay(PWMs)
    % Updates the thrust decay factor based on current duty cycles
    %
    % Inputs:
    %   PWMs - Current duty cycle values (vector)
    %
    % Outputs:
    %   thrust_decay_factor - Updated decay factor (scalar)
    %   count - Number of active thrusters (scalar)

    % Normalize PWMs if necessary
    if max(PWMs) > 1
        PWMs = PWMs / max(PWMs);
    end

    % Count active thrusters
    count = sum(PWMs > 0);
    
    % Compute average duty cycle for active thrusters
    average_duty_cycle_per_thruster = sum(max(PWMs, 0)) / max(count, 1);

    % Update thrust decay factor based on average duty cycle
    if average_duty_cycle_per_thruster < 0.3 || count == 0
        thrust_decay_factor = 1;
    else
        thrust_decay_factor = max(0.6 - 2 * average_duty_cycle_per_thruster + 1, 0.5);
    end
end

== matlab function spot410/Thruster Control Code/Change RED Behavior/Calculate Duty Cycle/Rotate Forces to Inertial/Create Rotation Matrix ==
  data: Rz input; C_Ib output
function C_Ib = RotateFrame(Rz)

C_bI = [  cos(Rz) sin(Rz)
         -sin(Rz) cos(Rz) ];

C_Ib = inv(C_bI);

end

== matlab function spot410/Thruster Control Code/Change RED Behavior/Rotate Forces to Body/Create Rotation Matrix ==
  data: Rz input; C_bI output
function C_bI = RotateFrame(Rz)

C_bI = [  cos(Rz) sin(Rz)
         -sin(Rz) cos(Rz) ];

end

== matlab function spot410/SpotGnc/SpotEstimator ==
  data: phase input; proc input; cmd input; est output; est_vel output; paramEst parameter; est_bias output; debug output
function [est,est_vel,est_bias,debug] = SpotEstimator(phase, proc, cmd, paramEst)

    [est,est_vel,est_bias,debug] = SpotEstimator(phase, proc, cmd, paramEst);

end

== matlab function spot410/Thruster Control Code/Change BLACK Behavior/Calculate Duty Cycle/MATLAB Function1 ==
  data: ThrustPer_Final output; ThrustPer input; PWMFreq parameter
function ThrustPer_Final  = ThrusterSat(ThrustPer, PWMFreq)

    ValveTime       = 0.007;
    TControl        = 1/PWMFreq;

    ThrustPer_Final = zeros(8,1);
    
    if max(ThrustPer) > 1
        ThrustPer_Sat = ThrustPer/max(ThrustPer);
    else
        ThrustPer_Sat = ThrustPer;
    end
    
    for i = 1:8
        if ThrustPer_Sat(i) > ValveTime/TControl 
            ThrustPer_Final(i) = ThrustPer_Sat(i);
        else
            ThrustPer_Final(i) = 0;
        end
    end


end

== matlab function spot410/Thruster Control Code/Change RED Behavior/Calculate Duty Cycle/MATLAB Function8 ==
  data: ThrustPer_Final output; ThrustPer input; PWMFreq parameter
function ThrustPer_Final  = ThrusterSat(ThrustPer, PWMFreq)

    ValveTime       = 0.007;
    TControl        = 1/PWMFreq;

    ThrustPer_Final = zeros(8,1);
    
    if max(ThrustPer) > 1
        ThrustPer_Sat = ThrustPer/max(ThrustPer);
    else
        ThrustPer_Sat = ThrustPer;
    end
    
    for i = 1:8
        if ThrustPer_Sat(i) > ValveTime/TControl 
            ThrustPer_Final(i) = ThrustPer_Sat(i);
        else
            ThrustPer_Final(i) = 0;
        end
    end


end

== matlab function spot410/SpotGnc/SpotRefGen ==
  data: phase input; t input; proc input; ref output; paramRefGen parameter; ref_vel output
function [ref,ref_vel] = SpotRefGen(phase, t, proc, paramRefGen)

    [ref,ref_vel] = SpotRefGen(phase, t, proc, paramRefGen);

end

== matlab function spot410/Simulate Plant Dynamics/RED and ARM Dynamics/RED + ARM/Dynamics Model ==
  data: q_dot output; x input; InertiaS input; CoriolisS input; u input; Gamma1_sh parameter; Gamma2_sh parameter; Gamma3_sh parameter; Gamma5_sh parameter; Gamma4_sh parameter; Gamma6_sh parameter; Gamma1_el parameter; Gamma2_el parameter; Gamma3_el parameter; Gamma5_el parameter; Gamma4_el parameter; Gamma6_el parameter; Gamma1_wr parameter; Gamma2_wr parameter; Gamma3_wr parameter; Gamma5_wr parameter; Gamma4_wr parameter; Gamma6_wr parameter; q_ddot output
function [q_dot, q_ddot]  = DynamicsModel(x, InertiaS, CoriolisS, u,...
    Gamma1_sh, Gamma2_sh, Gamma3_sh, Gamma5_sh, Gamma4_sh, Gamma6_sh,...
    Gamma1_el, Gamma2_el, Gamma3_el, Gamma5_el, Gamma4_el, Gamma6_el,...
    Gamma1_wr, Gamma2_wr, Gamma3_wr, Gamma5_wr, Gamma4_wr, Gamma6_wr)


    fqdot1 = Gamma1_sh*(tanh(Gamma2_sh*x(10)) - tanh(Gamma3_sh*x(10))) + Gamma4_sh*tanh(Gamma5_sh*x(10)) + Gamma6_sh*x(10);

    fqdot2 = Gamma1_el*(tanh(Gamma2_el*x(11)) - tanh(Gamma3_el*x(11))) + Gamma4_el*tanh(Gamma5_el*x(11)) + Gamma6_el*x(11);

    fqdot3 = Gamma1_wr*(tanh(Gamma2_wr*x(12)) - tanh(Gamma3_wr*x(12))) + Gamma4_wr*tanh(Gamma5_wr*x(12)) + Gamma6_wr*x(12);
    
    q_dot  = x(7:12);
    q_ddot = pinv(InertiaS)*(u - CoriolisS*x(7:12) - [0;0;0;fqdot1;fqdot2;fqdot3]);
    
end

== matlab function spot410/SpotGnc/MATLAB Function ==
  data: phase input; puckState output; armState output; paramFlag parameter
function [puckState,armState] = SpotFlag(phase, paramFlag)

    [puckState,armState] = SpotFlag(phase, paramFlag);

end

== matlab function spot410/SpotGnc/MATLAB Function1 ==
  data: t input; phase output; paramPhaseMgmt parameter
function phase  = SpotPhaseMgmt(t, paramPhaseMgmt)

    [phase] = SpotPhaseMgmt(t, paramPhaseMgmt);

end

== matlab function spot410/PhaseSpace Camera Code/Use Hardware to Obtain States/Receive and Process Phasespace Data/Check for Sychronization/MATLAB Function ==
  data: StartClock output; RedReceiving input; BlackReceiving input; BlueReceiving input; platformSelection parameter
function StartClock = CheckForSync(RedReceiving, BlackReceiving, BlueReceiving, platformSelection)
        
    StartClock = 0;
    
    if (platformSelection == 1)
        
        if RedReceiving == 1

            StartClock = 1;

        else

            StartClock = 0;

        end
        
    elseif (platformSelection == 2)
        
        if BlackReceiving == 1

            StartClock = 1;

        else

            StartClock = 0;

        end  
        
    elseif (platformSelection == 3)
        
        if RedReceiving == 1 && BlackReceiving == 1

            StartClock = 1;

        else

            StartClock = 0;

        end    
        
    elseif (platformSelection == 4)
        
        if RedReceiving == 1 && BlackReceiving == 1

            StartClock = 1;

        else

            StartClock = 0;

        end
        
    elseif (platformSelection == 5)
        
        if RedReceiving == 1

            StartClock = 1;

        else

            StartClock = 0;

        end
        
    elseif (platformSelection == 6)
        
        if BlueReceiving == 1

            StartClock = 1;

        else

            StartClock = 0;

        end
        
    elseif (platformSelection == 7)
        
        if RedReceiving == 1 && BlueReceiving == 1

            StartClock = 1;

        else

            StartClock = 0;

        end
        
    elseif (platformSelection == 8)
        
        if RedReceiving == 1 && BlackReceiving == 1 && BlueReceiving == 1

            StartClock = 1;

        else

            StartClock = 0;

        end
        
    elseif (platformSelection == 9)
        
        if BlackReceiving == 1 && BlueReceiving == 1

            StartClock = 1;

        else

            StartClock = 0;

        end
                           
    elseif (platformSelection == 10)
        
        if RedReceiving == 1 && BlueReceiving == 1

            StartClock = 1;

        else

            StartClock = 0;

        end
        
    elseif (platformSelection == 11)
        
        if RedReceiving == 1 && BlackReceiving == 1 && BlueReceiving == 1

            StartClock = 1;

        else

            StartClock = 0;

        end
        
    end



end

== matlab function spot410/Thruster Control Code/Change BLUE Behavior/Calculate Duty Cycle/MATLAB Function1 ==
  data: ThrustPer_Final output; ThrustPer input; PWMFreq parameter
function ThrustPer_Final  = ThrusterSat(ThrustPer, PWMFreq)

    ValveTime       = 0.007;
    TControl        = 1/PWMFreq;

    ThrustPer_Final = zeros(8,1);
    
    if max(ThrustPer) > 1
        ThrustPer_Sat = ThrustPer/max(ThrustPer);
    else
        ThrustPer_Sat = ThrustPer;
    end
    
    for i = 1:8
        if ThrustPer_Sat(i) > ValveTime/TControl 
            ThrustPer_Final(i) = ThrustPer_Sat(i);
        else
            ThrustPer_Final(i) = 0;
        end
    end


end

== matlab function spot410/3 - Control/Default LQR Control (RED)/Calculate Error/MATLAB Function ==
  data: Rz_path input; Rz_error output; Rz_measured input
function Rz_error = SmoothAngularDifference(Rz_path, Rz_measured)

    Rz_error = mod(Rz_measured-Rz_path+pi, 2*pi)-pi;


end

== matlab function spot410/3 - Control/Default LQR Control (BLACK)/Calculate Error/MATLAB Function ==
  data: Rz_path input; Rz_error output; Rz_measured input
function Rz_error = SmoothAngularDifference(Rz_path, Rz_measured)

    Rz_error = mod(Rz_measured-Rz_path+pi, 2*pi)-pi;


end

== matlab function spot410/3 - Control/Default PD Control (RED)/Calculate Error/MATLAB Function ==
  data: Rz_path input; Rz_error output; Rz_measured input
function Rz_error = SmoothAngularDifference(Rz_path, Rz_measured)

    Rz_error = mod(Rz_measured-Rz_path+pi, 2*pi)-pi;


end
